simulink model "tanques_2"  (R2021b)
settings: Solver=ode8  StartTime=0.0  StopTime=100.0  FixedStep=0.000002  RelTol=1e-3
settings Model: Creator=eless  LastModifiedBy=User

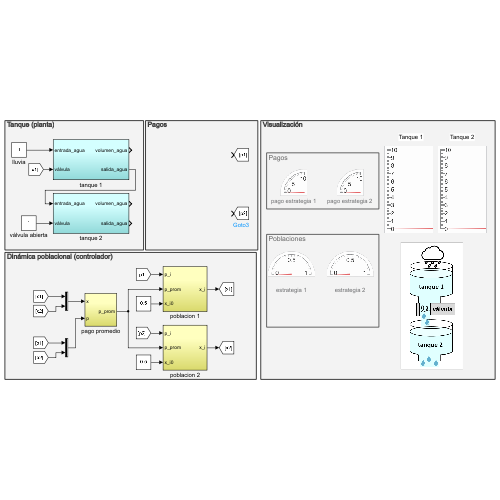
[thumbnail: Simulink's stored preview of the top-level diagram]
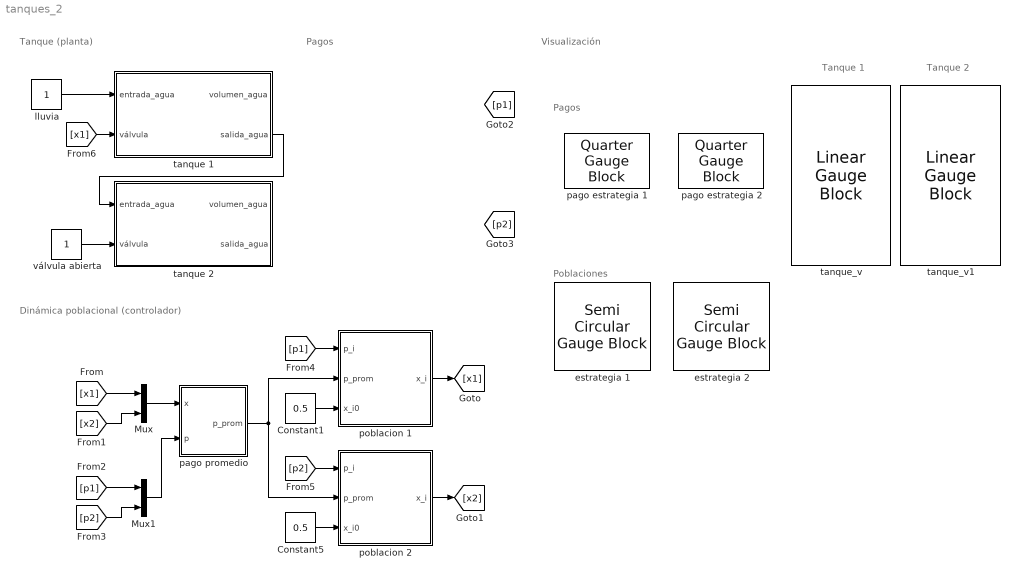
== system tanques_2 ==
  note: Tanque 1
  note: Poblaciones
  note: Pagos
  note: Visualización
  note: Tanque (planta)
  note: Dinámica poblacional (controlador)
  note: Pagos
  note: Tanque 2
  Constant1 : Constant  Value=0.5
  Constant5 : Constant  Value=0.5
  Mux : Mux  Inputs=2
  Mux1 : Mux  Inputs=2
  estrategia 1 : SemiCircularGaugeBlock  LabelPosition=Hide  ScaleMax=1  TickInterval=0.5
  estrategia 2 : SemiCircularGaugeBlock  LabelPosition=Hide  ScaleMax=1  TickInterval=0.5
  lluvia : Constant
  pago estrategia 1 : QuarterGaugeBlock  LabelPosition=Hide  ScaleMax=10
  pago estrategia 2 : QuarterGaugeBlock  LabelPosition=Hide  ScaleMax=10
  pago promedio : Subsystem
  poblacion 1 : Subsystem
  poblacion 2 : Subsystem
  tanque 1 : Subsystem
  tanque 2 : Subsystem
  tanque_v : LinearGaugeBlock  LabelPosition=Hide  ScaleMax=10
  tanque_v1 : LinearGaugeBlock  LabelPosition=Hide  ScaleMax=10
  válvula abierta : Constant
  wires:
  [x1] -> Mux/1
  [x2] -> Mux/2
  [p1] -> Mux1/1
  [p2] -> Mux1/2
  [p1] -> poblacion 1/1(p_i)
  poblacion 1/1(x_i) -> [x1]
  Constant1/1 -> poblacion 1/3(x_i0)
  poblacion 2/1(x_i) -> [x2]
  [p2] -> poblacion 2/1(p_i)
  Constant5/1 -> poblacion 2/3(x_i0)
  Mux/1 -> pago promedio/1(x)
  Mux1/1 -> pago promedio/2(p)
  lluvia/1 -> tanque 1/1(entrada_agua)
  [x1] -> tanque 1/2(válvula)
  pago promedio/1(p_prom) -> poblacion 2/2(p_prom), poblacion 1/2(p_prom)
  válvula abierta/1 -> tanque 2/2(válvula)
  tanque 1/2(salida_agua) -> tanque 2/1(entrada_agua)

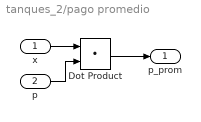
== system tanques_2/pago promedio ==
  x : Inport
  p : Inport  Port=2
  Dot Product : DotProduct  InputSameDT=on  OutDataTypeStr=Inherit: Inherit via internal rule
  p_prom : Outport
  wires:
  Dot Product/1 -> p_prom/1
  x/1 -> Dot Product/1
  p/1 -> Dot Product/2

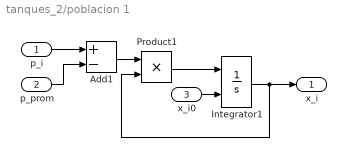
== system tanques_2/poblacion 1 ==
  p_i : Inport
  p_prom : Inport  Port=2
  x_i0 : Inport  Port=3
  Add1 : Sum  Inputs=+-
  Integrator1 : Integrator  InitialConditionSource=external  InitialCondition=0.5
  Product1 : Product
  x_i : Outport
  wires:
  Add1/1 -> Product1/1
  Integrator1/1 -> x_i/1, Product1/2
  Product1/1 -> Integrator1/1
  p_i/1 -> Add1/1
  p_prom/1 -> Add1/2
  x_i0/1 -> Integrator1/2

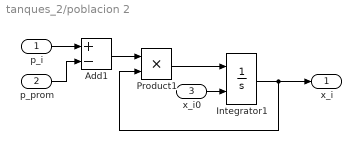
== system tanques_2/poblacion 2 ==
  p_i : Inport
  p_prom : Inport  Port=2
  x_i0 : Inport  Port=3
  Add1 : Sum  Inputs=+-
  Integrator1 : Integrator  InitialConditionSource=external  InitialCondition=0.5
  Product1 : Product
  x_i : Outport
  wires:
  x_i0/1 -> Integrator1/2
  p_prom/1 -> Add1/2
  p_i/1 -> Add1/1
  Product1/1 -> Integrator1/1
  Integrator1/1 -> x_i/1, Product1/2
  Add1/1 -> Product1/1

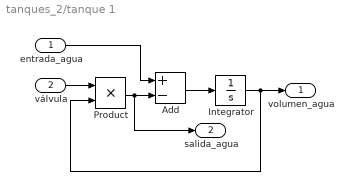
== system tanques_2/tanque 1 ==
  entrada_agua : Inport
  válvula : Inport  Port=2
  Add : Sum  Inputs=+-
  Integrator : Integrator  InitialCondition=9
  Product : Product
  volumen_agua : Outport
  salida_agua : Outport  Port=2
  wires:
  Product/1 -> Add/2, salida_agua/1
  Add/1 -> Integrator/1
  Integrator/1 -> volumen_agua/1, Product/2
  válvula/1 -> Product/1
  entrada_agua/1 -> Add/1

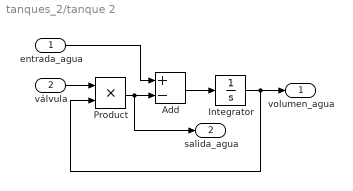
== system tanques_2/tanque 2 ==
  entrada_agua : Inport
  válvula : Inport  Port=2
  Add : Sum  Inputs=+-
  Integrator : Integrator  InitialCondition=2
  Product : Product
  volumen_agua : Outport
  salida_agua : Outport  Port=2
  wires:
  entrada_agua/1 -> Add/1
  válvula/1 -> Product/1
  Integrator/1 -> Product/2, volumen_agua/1
  Add/1 -> Integrator/1
  Product/1 -> salida_agua/1, Add/2
